simulink model "SiemensBike"  (R2025b)
settings: Solver=ode14x  StartTime=0  StopTime=inf  FixedStep=.01  RelTol=1e-2  EnableMultiTasking=on
StopFcn:
  | %toc
undefined symbols (not defined in the file): CtrlTcuInitGear, EnvAbsPrs, EnvAirTemp, EnvNomFrictionScaling, EnvNominalGrade, EnvWindVelX, EnvWindVelY, EnvWindVelZ, MotoFrmLngth, Sim3dSensor
libraries: vehdynlibviscommon x3, sim3dgroundtruthsensorlib x2, simulink x1, sharedtransform x1, autolibutils x1
(part 3 of 3)

== system SiemensBike/Environment/Ground Feedback/3D Engine/3D Engine Source/Single Point ==
  Bus Creator1 : BusCreator  Inputs=2
  Bus Selector2 : BusSelector  OutputSignals=Wheel1Positions,Wheel2Positions
  Constant2 : Constant  Value=repmat(eye(3),1,1,2)  SampleTime=-1
  Data Type Conversion1 : DataTypeConversion  SaturateOnIntegerOverflow=off  RndMeth=Floor
  Data Type Conversion2 : DataTypeConversion  SaturateOnIntegerOverflow=off  RndMeth=Floor
  First Order Hold5 : FirstOrderHold  ErrorTolerance=1
  First Order Hold6 : FirstOrderHold  ErrorTolerance=1
  Range Limiter5 : Saturate  UpperLimit=1e3  LowerLimit=-1e3  ZeroCross=off
  Range Limiter6 : Saturate  UpperLimit=1e3  LowerLimit=-1e3  ZeroCross=off
  Signal Specification6 : SignalSpecification  Unit=m
  Signal Specification7 : SignalSpecification  Unit=m
  Simulation 3D Terrain Sensor1 : sim3dgroundtruthsensorlib/Simulation 3D Terrain Sensor  Priority=1  vehTagList={'Scene Origin';'SimulinkVehicle1'}  sensorTag=Sim3dSensor�  sensorId=1  sensorName=Sim3dSensor�  vehTag=SimulinkVehicle1  CoordinateSystem=Default  tmountOffset=[0, 0, 0]  rmountOffset=[0,0,0,]  RayOrigins=[0 0 1]  RayDirections=[0 0 -1]  RayLengths=20  NumberOfWheels=2  VisualizeTraceLines=off  SampleTime=-1  aMode=2  ID=1
  Zend Select1 : Selector  NumberOfDimensions=2  InputPortWidth=3  IndexOptions=Select all,Index vector (dialog)  Indices=[1 3],3  OutputSizes=1,1
  Zend Select2 : Selector  NumberOfDimensions=2  InputPortWidth=3  IndexOptions=Select all,Index vector (dialog)  Indices=[1 3],3  OutputSizes=1,1
  z : Outport
  DCM : Outport  Port=2
  wires:
  Constant2/1 -> DCM/1  "DCM"
  Bus Creator1/1 -> z/1  "z"
  Range Limiter5/1 -> Zend Select1/1
  First Order Hold5/1 -> Signal Specification6/1
  Bus Selector2/1 -> Range Limiter5/1  "<Wheel1Positions>"
  Data Type Conversion1/1 -> First Order Hold5/1
  Range Limiter6/1 -> Zend Select2/1
  Data Type Conversion2/1 -> First Order Hold6/1
  Zend Select2/1 -> Data Type Conversion2/1
  First Order Hold6/1 -> Signal Specification7/1
  Bus Selector2/2 -> Range Limiter6/1  "<Wheel2Positions>"
  Signal Specification7/1 -> Bus Creator1/2  "G_R_z"
  Zend Select1/1 -> Data Type Conversion1/1
  Simulation 3D Terrain Sensor1/1 -> Bus Selector2/1
  Signal Specification6/1 -> Bus Creator1/1  "G_F_z"

== system SiemensBike/Environment/Ground Feedback/3D Engine/3D Engine Source/Multiple Points/For Each Subsystem ==
  phi,theta,psi : Inport  Partition=on  PartitionDimension=2  PartitionWidth=1  PartitionOffset=0
  For Each : ForEach  DisableCoverage=on
  Rotation Angles to Direction Cosine Matrix1 : sharedtransform/Rotation Angles to Direction Cosine Matrix  rotationOrder=YXZ  aMode=2
  Selector5 : Selector  InputPortWidth=3  IndexOptions=Index vector (dialog)  Indices=[2 1 3]  OutputSizes=1
  WheelDCM : Outport  ConcatenationDimension=3
  wires:
  phi,theta,psi/1 -> Selector5/1
  Rotation Angles to Direction Cosine Matrix1/1 -> WheelDCM/1
  Selector5/1 -> Rotation Angles to Direction Cosine Matrix1/1

== matlab function SiemensBike/Server Communication/UDPSend ==
  data: engspeed input; angspeed input; temp input; emissions input
function sendData(engspeed, angspeed, temp, emissions)
    % 1. TELL SIMULINK TO USE MATLAB ENGINE (Fixes the Code Gen Error)
    coder.extrinsic('udpport', 'write', 'sprintf', 'pi');
    
    % persistent variable to keep the UDP object open between steps
    persistent udpsend;
    
    % 2. INITIALIZE THE PORT
    if isempty(udpsend) 
        % LocalPort 5006 sends TO the Java Server on 5005
        udpsend = udpport("LocalPort", 5006); 
    end
    
    % 3. CALCULATE RPM
    % Using 9.5493 as the conversion factor (60 / 2*pi)
    rpm = angspeed * 60 / (2 * pi);
    
    % 4. FORMAT THE BIG STRING
    % Example output: "5500.00,85.50,92.10,0.04"
    dataString = sprintf('%.2f,%.2f,%.2f,%.2f', rpm, engspeed, temp, emissions);
    
    % 5. SEND TO JAVA
    % "char" ensures Java reads standard ASCII/UTF-8 bytes
    write(udpsend, dataString, "char", "127.0.0.1", 5005);
    
end

== matlab function SiemensBike/Visualization/Excessive Roll Angle Detection ==
  data: phi input; stopSim output
function stopSim = phiStop(phi)
%#codegen

% Initialize output
stopSim = false;

% Check the condition
rollLim = pi/3;
if abs(phi)>=rollLim
    % Display a warning message    
    warning(message('vdynblks:vehdynErrMsg:excessivePhi',num2str(rad2deg(rollLim))));
    % Set output to indicate a warning has been triggered
    stopSim = true;
end
